simulink subsystem "ServoValveLinkage"  (R2020b)
settings: Solver=VariableStepAuto  StartTime=0.0  StopTime=10.0  RelTol=1e-3
model mask{servoValveSignConvention=ServoValveSignConvention.POSITIVE_AWAY_FROM_VALVE, valveCloseHandleRotationDirection=ValveCloseHandleRotationDirection.AWAY_FROM_SERVO, g=21, a=10.17, h=30.625, b=20.78, linkageServoAngleForClosedDegrees=217, servoCommandedCloseAngleDegrees=0}
  mask prompts: servoValveSignConvention "Servo valve sign convention"; valveCloseHandleRotationDirection "Valve handle close direction"; g "Distance between pivots (mm)"; a "Length of crank arm (mm)"; h "Length of coupler arm (mm)"; b "Length of rocket arm (mm)"; linkageServoAngleForClosedDegrees "Servo angle for closed valve degrees (in linkage angle convention)"; servoCommandedCloseAngleDegrees "Angle to command to servo for closed valve degrees"
undefined symbols (not defined in the file or in its folder): linkageValveAngleForOpenDegrees
settings Model: Creator=Edward  LastModifiedBy=Edward

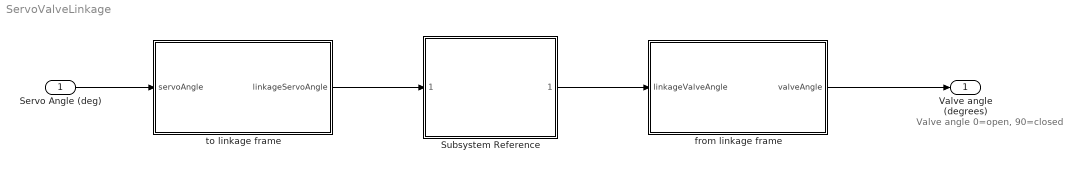
== system ServoValveLinkage ==
  note: Valve angle 0=open, 90=closed
  Servo Angle (deg) : Inport
  Subsystem Reference : Subsystem  ReferencedSubsystem=AnalyticFourBarLinkage  g=g  a=a  h=h  b=b  solutionSelector=1
  from linkage frame : MATLAB Function  TreatAsAtomicUnit=on
  to linkage frame : MATLAB Function  TreatAsAtomicUnit=on
  Valve angle (degrees) : Outport
  wires:
  Servo Angle (deg)/1 -> to linkage frame/1(servoAngle)
  to linkage frame/1(linkageServoAngle) -> Subsystem Reference/1
  Subsystem Reference/1 -> from linkage frame/1(linkageValveAngle)
  from linkage frame/1(valveAngle) -> Valve angle (degrees)/1

== matlab function ServoValveLinkage/to linkage frame ==
  data: servoAngle input; linkageServoAngle output; linkageServoAngleForClosedDegrees parameter; servoCommandedCloseAngleDegrees parameter; servoValveSignConvention parameter Enum: ServoValveSignConvention; valveCloseHandleRotationDirection parameter Enum: ValveCloseHandleRotationDirection
function linkageServoAngle = fcn(servoAngle, linkageServoAngleForClosedDegrees, ...
servoCommandedCloseAngleDegrees, servoValveSignConvention, valveCloseHandleRotationDirection)
%Get servo angle in linkage coordinate system from actual servoAngle
if(servoValveSignConvention == ServoValveSignConvention.POSITIVE_AWAY_FROM_VALVE)
    if(valveCloseHandleRotationDirection == ValveCloseHandleRotationDirection.TOWARDS_SERVO)
        linkageServoAngle = clampDegreeAngle(servoAngle-linkageServoAngleForClosedDegrees-servoCommandedCloseAngleDegrees);
        return;
    elseif(valveCloseHandleRotationDirection == ValveCloseHandleRotationDirection.AWAY_FROM_SERVO)
        linkageServoAngle = clampDegreeAngle(-(servoAngle-linkageServoAngleForClosedDegrees)-servoCommandedCloseAngleDegrees);
        return;
    end
elseif (servoValveSignConvention == ServoValveSignConvention.POSITIVE_TOWARDS_VALVE)
    if(valveCloseHandleRotationDirection == ValveCloseHandleRotationDirection.TOWARDS_SERVO)
        linkageServoAngle = clampDegreeAngle(-servoAngle + servoCommandedCloseAngleDegrees + linkageServoAngleForClosedDegrees);
        return;
    elseif(valveCloseHandleRotationDirection == ValveCloseHandleRotationDirection.AWAY_FROM_SERVO)
        linkageServoAngle = clampDegreeAngle(servoAngle+linkageServoAngleForClosedDegrees-servoCommandedCloseAngleDegrees);
        return;
    end
end
linkageServoAngle = -1;

== matlab function ServoValveLinkage/from linkage frame ==
  data: linkageValveAngle input; valveAngle output; linkageValveAngleForOpenDegrees parameter; valveCloseHandleRotationDirection parameter Enum: ValveCloseHandleRotationDirection
function valveAngle = fcn(linkageValveAngle, linkageValveAngleForOpenDegrees, ...
    valveCloseHandleRotationDirection)
%Get actual valve angle (0=open,90=closed) from linkage coordinate system
valveAngle = -1;
if(valveCloseHandleRotationDirection == ValveCloseHandleRotationDirection.TOWARDS_SERVO)
    valveAngle = clampDegreeAngle(linkageValveAngle-linkageValveAngleForOpenDegrees);
elseif(valveCloseHandleRotationDirection == ValveCloseHandleRotationDirection.AWAY_FROM_SERVO)
    valveAngle = clampDegreeAngle(-linkageValveAngle-linkageValveAngleForOpenDegrees);
end
if(valveAngle < 0 || valveAngle > 300)
   valveAngle = 0; 
end
if(valveAngle > 90 && valveAngle < 100)
   valveAngle = 90; 
end
